simulink model "Robocon_mark1_1"  (R2020b)
settings: Solver=ode45  StartTime=0.0  StopTime=10.0  MaxStep=1e-2  RelTol=1e-4  AbsTol=1e-5  EnableMultiTasking=on
values from neighbouring files (symbols this model uses):
  arena_breadth = 10    [Robocon_DataFile.m]
  arena_length = 13.3    [Robocon_DataFile.m]
undefined symbols (not defined in the file or in its folder): DiscIntNeverNeededParam, sigbuilder_block, smiData, X, Y, Z
libraries: sm_lib x232, Contact_Forces_Lib x55, nesl_utility x9, mobileRoboticsLib x4, simulink_extras x2, fl_lib x1
(part 6 of 6)

== system Robocon_mark1_1/TR ROBOT/CONTACT FORCE/PLATE CONTACT4 ==
  Sphere to Plane Force : Contact_Forces_Lib/3D/Sphere to Plane Force  sphere_rad=rugby_main  plane_lenx=0.16  plane_leny=0.191  plane_depth=0  force_law=Linear  k_contact=1e4  b_contact=1e2  pen_full_damp_F=1e-4  pen_exponent=1  custom_param_1=1  custom_param_2=1  friction_law=Stick-Slip Continuous  mu_kinetic=0.5  mu_static=0.7  v_thr=0.001  vis_on=off  vis_opc_en=0  vis_len_plaBz=0.005  vis_clr=[0.9 0.2 0.2]  vis_opc=0.7
  Terminator1 : Terminator
  MIDDLE : PMIOPort  Side=Left
  TO PLATE : PMIOPort  Port=2  Side=Right
  wires:
  Sphere to Plane Force/1 -> Terminator1/1
  connections:
  TO PLATE/RConn1 -- Sphere to Plane Force/RConn1
  Sphere to Plane Force/LConn1 -- MIDDLE/RConn1

== system Robocon_mark1_1/TR ROBOT/CONTACT FORCE/PLATE CONTACT5 ==
  Sphere to Plane Force : Contact_Forces_Lib/3D/Sphere to Plane Force  sphere_rad=rugby_main  plane_lenx=0.16  plane_leny=0.097  plane_depth=0  force_law=Linear  k_contact=1e4  b_contact=1e2  pen_full_damp_F=1e-4  pen_exponent=1  custom_param_1=1  custom_param_2=1  friction_law=Stick-Slip Continuous  mu_kinetic=0.5  mu_static=0.7  v_thr=0.001  vis_on=off  vis_opc_en=0  vis_len_plaBz=0.005  vis_clr=[0.9 0.2 0.2]  vis_opc=0.7
  Sphere to Plane Force1 : Contact_Forces_Lib/3D/Sphere to Plane Force  sphere_rad=rugby_middle_lower  plane_lenx=0.16  plane_leny=0.097  plane_depth=0  force_law=Linear  k_contact=1e4  b_contact=1e2  pen_full_damp_F=1e-4  pen_exponent=1  custom_param_1=1  custom_param_2=1  friction_law=Stick-Slip Continuous  mu_kinetic=0.5  mu_static=0.7  v_thr=0.001  vis_on=off  vis_opc_en=0  vis_len_plaBz=0.005  vis_clr=[0.9 0.2 0.2]  vis_opc=0.7
  Sphere to Plane Force2 : Contact_Forces_Lib/3D/Sphere to Plane Force  sphere_rad=rugby_middle_upper  plane_lenx=0.16  plane_leny=0.097  plane_depth=0  force_law=Linear  k_contact=1e4  b_contact=1e2  pen_full_damp_F=1e-4  pen_exponent=1  custom_param_1=1  custom_param_2=1  friction_law=Stick-Slip Continuous  mu_kinetic=0.5  mu_static=0.7  v_thr=0.001  vis_on=off  vis_opc_en=0  vis_len_plaBz=0.005  vis_clr=[0.9 0.2 0.2]  vis_opc=0.7
  Terminator : Terminator
  Terminator1 : Terminator
  Terminator2 : Terminator
  "UPPER " : PMIOPort  Side=Left
  MIDDLE : PMIOPort  Port=2  Side=Left
  TO PLATE : PMIOPort  Port=3  Side=Right
  LOWER : PMIOPort  Port=4  Side=Left
  wires:
  Sphere to Plane Force2/1 -> Terminator/1
  Sphere to Plane Force1/1 -> Terminator2/1
  Sphere to Plane Force/1 -> Terminator1/1
  connections:
  Sphere to Plane Force/LConn1 -- MIDDLE/RConn1
  Sphere to Plane Force1/LConn1 -- LOWER/RConn1
  Sphere to Plane Force2/LConn1 -- "UPPER "/RConn1
  TO PLATE/RConn1 -- Sphere to Plane Force2/RConn1 -- Sphere to Plane Force/RConn1 -- Sphere to Plane Force1/RConn1

== system Robocon_mark1_1/TR ROBOT/CONTACT FORCE/ROUND PLATE CONTACT ==
  Sphere to Tube Force : Contact_Forces_Lib/3D/Sphere to Tube Force  radius_sphere=rugby_middle_upper  radius_tube=0.188  d_tube=0.01  l_tube=0.16  active_angle=[-27 87]  force_law=Linear  k_contact=1e6  b_contact=1e2  pen_full_damp_F=1e-4  pen_exponent=1  custom_param_1=1  custom_param_2=1  friction_law=Stick-Slip Continuous  mu_kinetic=0.5  mu_static=0.7  v_thr=0.001  vis_on=off  vis_opc_en=0  vis_len_tubBx=0.225*0.02  vis_clr=[0.9 0.2 0.2]  vis_opc=0.7
      settings: SourceProductName=Simscape Multibody Contact Forces Library
  Sphere to Tube Force1 : Contact_Forces_Lib/3D/Sphere to Tube Force  radius_sphere=rugby_main  radius_tube=0.188  d_tube=0.01  l_tube=0.16  active_angle=[-27 87]  force_law=Linear  k_contact=1e3  b_contact=1e2  pen_full_damp_F=1e-4  pen_exponent=1  custom_param_1=1  custom_param_2=1  friction_law=Stick-Slip Continuous  mu_kinetic=0.5  mu_static=0.7  v_thr=0.001  vis_on=off  vis_opc_en=0  vis_len_tubBx=0.225*0.02  vis_clr=[0.9 0.2 0.2]  vis_opc=0.7
      settings: SourceProductName=Simscape Multibody Contact Forces Library
  Sphere to Tube Force2 : Contact_Forces_Lib/3D/Sphere to Tube Force  radius_sphere=rugby_middle_lower  radius_tube=0.188  d_tube=0.01  l_tube=0.16  active_angle=[-27 87]  force_law=Linear  k_contact=1e6  b_contact=1e2  pen_full_damp_F=1e-4  pen_exponent=1  custom_param_1=1  custom_param_2=1  friction_law=Stick-Slip Continuous  mu_kinetic=0.5  mu_static=0.7  v_thr=0.001  vis_on=off  vis_opc_en=0  vis_len_tubBx=0.225*0.02  vis_clr=[0.9 0.2 0.2]  vis_opc=0.7
      settings: SourceProductName=Simscape Multibody Contact Forces Library
  Terminator : Terminator
  Terminator1 : Terminator
  Terminator2 : Terminator
  "UPPER " : PMIOPort  Side=Left
  MIDDLE : PMIOPort  Port=2  Side=Left
  TO PLATE : PMIOPort  Port=3  Side=Right
  LOWER : PMIOPort  Port=4  Side=Left
  wires:
  Sphere to Tube Force1/1 -> Terminator1/1
  Sphere to Tube Force2/1 -> Terminator2/1
  Sphere to Tube Force/1 -> Terminator/1
  connections:
  Sphere to Tube Force/RConn1 -- TO PLATE/RConn1 -- Sphere to Tube Force1/RConn1 -- Sphere to Tube Force2/RConn1
  "UPPER "/RConn1 -- Sphere to Tube Force/LConn1
  Sphere to Tube Force2/LConn1 -- LOWER/RConn1
  Sphere to Tube Force1/LConn1 -- MIDDLE/RConn1

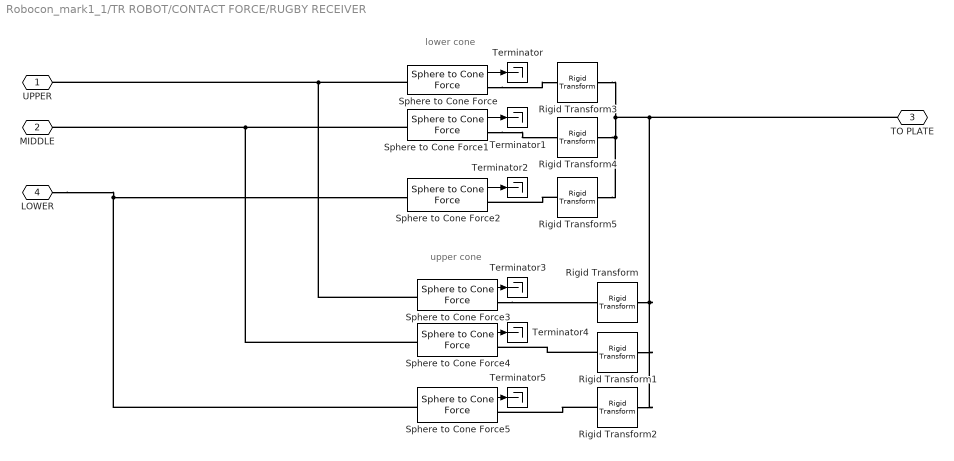
== system Robocon_mark1_1/TR ROBOT/CONTACT FORCE/RUGBY RECEIVER ==
  note: lower cone
  note: upper cone
  Rigid Transform : sm_lib/Frames and Transforms/Rigid Transform  TranslationMethod=StandardAxis  TranslationStandardOffset=710  TranslationLengthUnit=mm  TranslationStandardAxis=-Z  TranslationCartesianOffset=[0 0 0]  TranslationROffset=0  TranslationROffsetUnits=m  TranslationZOffset=0  TranslationZOffsetUnits=m  TranslationThetaOffset=0  TranslationThetaOffsetUnits=deg  RotationMethod=StandardAxis  RotationAngleUnits=deg  RotationStandardAxis=+Z  RotationAngle=-30  RotationArbitraryAxis=[0 0 1]  FollAlignAxisA=+X  BaseAlignAxisA=+Y  FollAlignAxisB=+Y  BaseAlignAxisB=+Z  RotationSequenceAxes=FollowerAxes  RotationSequence=XYX  RotationSequenceAngles=[0 0 0]  RotationSequenceAnglesUnits=deg  RotationMatrix=[1 0 0; 0 1 0; 0 0 1]
  Rigid Transform1 : sm_lib/Frames and Transforms/Rigid Transform  TranslationMethod=StandardAxis  TranslationStandardOffset=710  TranslationLengthUnit=mm  TranslationStandardAxis=-Z  TranslationCartesianOffset=[0 0 0]  TranslationROffset=0  TranslationROffsetUnits=m  TranslationZOffset=0  TranslationZOffsetUnits=m  TranslationThetaOffset=0  TranslationThetaOffsetUnits=deg  RotationMethod=StandardAxis  RotationAngleUnits=deg  RotationStandardAxis=+Z  RotationAngle=-30  RotationArbitraryAxis=[0 0 1]  FollAlignAxisA=+X  BaseAlignAxisA=+Y  FollAlignAxisB=+Y  BaseAlignAxisB=+Z  RotationSequenceAxes=FollowerAxes  RotationSequence=XYX  RotationSequenceAngles=[0 0 0]  RotationSequenceAnglesUnits=deg  RotationMatrix=[1 0 0; 0 1 0; 0 0 1]
  Rigid Transform2 : sm_lib/Frames and Transforms/Rigid Transform  TranslationMethod=StandardAxis  TranslationStandardOffset=710  TranslationLengthUnit=mm  TranslationStandardAxis=-Z  TranslationCartesianOffset=[0 0 0]  TranslationROffset=0  TranslationROffsetUnits=m  TranslationZOffset=0  TranslationZOffsetUnits=m  TranslationThetaOffset=0  TranslationThetaOffsetUnits=deg  RotationMethod=StandardAxis  RotationAngleUnits=deg  RotationStandardAxis=+Z  RotationAngle=-30  RotationArbitraryAxis=[0 0 1]  FollAlignAxisA=+X  BaseAlignAxisA=+Y  FollAlignAxisB=+Y  BaseAlignAxisB=+Z  RotationSequenceAxes=FollowerAxes  RotationSequence=XYX  RotationSequenceAngles=[0 0 0]  RotationSequenceAnglesUnits=deg  RotationMatrix=[1 0 0; 0 1 0; 0 0 1]
  Rigid Transform3 : sm_lib/Frames and Transforms/Rigid Transform  TranslationMethod=StandardAxis  TranslationStandardOffset=345  TranslationLengthUnit=mm  TranslationStandardAxis=-Z  TranslationCartesianOffset=[0 0 0]  TranslationROffset=0  TranslationROffsetUnits=m  TranslationZOffset=0  TranslationZOffsetUnits=m  TranslationThetaOffset=0  TranslationThetaOffsetUnits=deg  RotationMethod=StandardAxis  RotationAngleUnits=deg  RotationStandardAxis=+Z  RotationAngle=150  RotationArbitraryAxis=[0 0 1]  FollAlignAxisA=+X  BaseAlignAxisA=+Y  FollAlignAxisB=+Y  BaseAlignAxisB=+Z  RotationSequenceAxes=FollowerAxes  RotationSequence=XYX  RotationSequenceAngles=[0 0 0]  RotationSequenceAnglesUnits=deg  RotationMatrix=[1 0 0; 0 1 0; 0 0 1]
  Rigid Transform4 : sm_lib/Frames and Transforms/Rigid Transform  TranslationMethod=StandardAxis  TranslationStandardOffset=345  TranslationLengthUnit=mm  TranslationStandardAxis=-Z  TranslationCartesianOffset=[0 0 0]  TranslationROffset=0  TranslationROffsetUnits=m  TranslationZOffset=0  TranslationZOffsetUnits=m  TranslationThetaOffset=0  TranslationThetaOffsetUnits=deg  RotationMethod=StandardAxis  RotationAngleUnits=deg  RotationStandardAxis=+Z  RotationAngle=150  RotationArbitraryAxis=[0 0 1]  FollAlignAxisA=+X  BaseAlignAxisA=+Y  FollAlignAxisB=+Y  BaseAlignAxisB=+Z  RotationSequenceAxes=FollowerAxes  RotationSequence=XYX  RotationSequenceAngles=[0 0 0]  RotationSequenceAnglesUnits=deg  RotationMatrix=[1 0 0; 0 1 0; 0 0 1]
  Rigid Transform5 : sm_lib/Frames and Transforms/Rigid Transform  TranslationMethod=StandardAxis  TranslationStandardOffset=345  TranslationLengthUnit=mm  TranslationStandardAxis=-Z  TranslationCartesianOffset=[0 0 0]  TranslationROffset=0  TranslationROffsetUnits=m  TranslationZOffset=0  TranslationZOffsetUnits=m  TranslationThetaOffset=0  TranslationThetaOffsetUnits=deg  RotationMethod=StandardAxis  RotationAngleUnits=deg  RotationStandardAxis=+Z  RotationAngle=150  RotationArbitraryAxis=[0 0 1]  FollAlignAxisA=+X  BaseAlignAxisA=+Y  FollAlignAxisB=+Y  BaseAlignAxisB=+Z  RotationSequenceAxes=FollowerAxes  RotationSequence=XYX  RotationSequenceAngles=[0 0 0]  RotationSequenceAnglesUnits=deg  RotationMatrix=[1 0 0; 0 1 0; 0 0 1]
  Sphere to Cone Force : Contact_Forces_Lib/3D/Sphere to Cone Force  radius_sphere=rugby_middle_upper  cone_or=0.2  cone_ir=0.2  cone_theta=80  cone_h=0.345  active_angle=[-90 90]  d_cone=0  r_cone=0  cosConeTh=0  sinConeTh=0  force_law=Linear  k_contact=1e3  b_contact=100  pen_full_damp_F=1e-4  pen_exponent=1  custom_param_1=1  custom_param_2=1  friction_law=Stick-Slip Continuous  mu_kinetic=0.5  mu_static=0.7  v_thr=0.001  vis_on=off  vis_opc_en=0  vis_depth_conBx=0.02  vis_clr=[0.9 0.2 0.2]  vis_opc=0.7
      settings: SourceProductName=Simscape Multibody Contact Forces Library
  Sphere to Cone Force1 : Contact_Forces_Lib/3D/Sphere to Cone Force  radius_sphere=rugby_main  cone_or=0.2  cone_ir=0.2  cone_theta=80  cone_h=0.345  active_angle=[-90 90]  d_cone=0  r_cone=0  cosConeTh=0  sinConeTh=0  force_law=Linear  k_contact=1e3  b_contact=100  pen_full_damp_F=1e-4  pen_exponent=1  custom_param_1=1  custom_param_2=1  friction_law=Stick-Slip Continuous  mu_kinetic=0.5  mu_static=0.7  v_thr=0.001  vis_on=off  vis_opc_en=0  vis_depth_conBx=0.02  vis_clr=[0.9 0.2 0.2]  vis_opc=0.7
      settings: SourceProductName=Simscape Multibody Contact Forces Library
  Sphere to Cone Force2 : Contact_Forces_Lib/3D/Sphere to Cone Force  radius_sphere=rugby_middle_lower  cone_or=0.2  cone_ir=0.2  cone_theta=80  cone_h=0.345  active_angle=[-90 90]  d_cone=0  r_cone=0  cosConeTh=0  sinConeTh=0  force_law=Linear  k_contact=1e3  b_contact=1e2  pen_full_damp_F=1e-4  pen_exponent=1  custom_param_1=1  custom_param_2=1  friction_law=Stick-Slip Continuous  mu_kinetic=0.5  mu_static=0.7  v_thr=0.001  vis_on=off  vis_opc_en=0  vis_depth_conBx=0.02  vis_clr=[0.9 0.2 0.2]  vis_opc=0.7
      settings: SourceProductName=Simscape Multibody Contact Forces Library
  Sphere to Cone Force3 : Contact_Forces_Lib/3D/Sphere to Cone Force  radius_sphere=rugby_middle_upper  cone_or=0.27  cone_ir=0.27  cone_theta=80  cone_h=0.71  active_angle=[-90 90]  d_cone=0  r_cone=0  cosConeTh=0  sinConeTh=0  force_law=Linear  k_contact=1e3  b_contact=1e2  pen_full_damp_F=1e-4  pen_exponent=1  custom_param_1=1  custom_param_2=1  friction_law=Stick-Slip Continuous  mu_kinetic=0.5  mu_static=0.7  v_thr=0.001  vis_on=off  vis_opc_en=0  vis_depth_conBx=0.02  vis_clr=[0.9 0.2 0.2]  vis_opc=0.7
      settings: SourceProductName=Simscape Multibody Contact Forces Library
  Sphere to Cone Force4 : Contact_Forces_Lib/3D/Sphere to Cone Force  radius_sphere=rugby_main  cone_or=0.27  cone_ir=0.27  cone_theta=80  cone_h=0.71  active_angle=[-90 90]  d_cone=0  r_cone=0  cosConeTh=0  sinConeTh=0  force_law=Linear  k_contact=1e3  b_contact=1e2  pen_full_damp_F=1e-4  pen_exponent=1  custom_param_1=1  custom_param_2=1  friction_law=Stick-Slip Continuous  mu_kinetic=0.5  mu_static=0.7  v_thr=0.001  vis_on=off  vis_opc_en=0  vis_depth_conBx=0.02  vis_clr=[0.9 0.2 0.2]  vis_opc=0.7
      settings: SourceProductName=Simscape Multibody Contact Forces Library
  Sphere to Cone Force5 : Contact_Forces_Lib/3D/Sphere to Cone Force  radius_sphere=rugby_middle_lower  cone_or=0.27  cone_ir=0.27  cone_theta=80  cone_h=0.71  active_angle=[-90 90]  d_cone=0  r_cone=0  cosConeTh=0  sinConeTh=0  force_law=Linear  k_contact=1e3  b_contact=1e2  pen_full_damp_F=1e-4  pen_exponent=1  custom_param_1=1  custom_param_2=1  friction_law=Stick-Slip Continuous  mu_kinetic=0.5  mu_static=0.7  v_thr=0.001  vis_on=off  vis_opc_en=0  vis_depth_conBx=0.02  vis_clr=[0.9 0.2 0.2]  vis_opc=0.7
      settings: SourceProductName=Simscape Multibody Contact Forces Library
  Terminator{,1..5} (6 alike) : Terminator
  "UPPER " : PMIOPort  Side=Left
  MIDDLE : PMIOPort  Port=2  Side=Left
  TO PLATE : PMIOPort  Port=3  Side=Right
  LOWER : PMIOPort  Port=4  Side=Left
  wires:
  Sphere to Cone Force/1 -> Terminator/1
  Sphere to Cone Force2/1 -> Terminator2/1
  Sphere to Cone Force1/1 -> Terminator1/1
  Sphere to Cone Force3/1 -> Terminator3/1
  Sphere to Cone Force4/1 -> Terminator4/1
  Sphere to Cone Force5/1 -> Terminator5/1
  connections:
  Sphere to Cone Force1/LConn1 -- Sphere to Cone Force4/LConn1 -- MIDDLE/RConn1
  LOWER/RConn1 -- Sphere to Cone Force5/LConn1 -- Sphere to Cone Force2/LConn1
  Sphere to Cone Force/LConn1 -- Sphere to Cone Force3/LConn1 -- "UPPER "/RConn1
  Sphere to Cone Force3/RConn1 -- Rigid Transform/RConn1
  Rigid Transform2/RConn1 -- Sphere to Cone Force5/RConn1
  Rigid Transform1/RConn1 -- Sphere to Cone Force4/RConn1
  Rigid Transform/LConn1 -- Rigid Transform1/LConn1 -- Rigid Transform2/LConn1 -- Rigid Transform3/LConn1 -- Rigid Transform5/LConn1 -- Rigid Transform4/LConn1 -- TO PLATE/RConn1
  Sphere to Cone Force/RConn1 -- Rigid Transform3/RConn1
  Sphere to Cone Force1/RConn1 -- Rigid Transform4/RConn1
  Rigid Transform5/RConn1 -- Sphere to Cone Force2/RConn1

== system Robocon_mark1_1/TR ROBOT/trleftgripper_1_RIGID1/Signal Builder ==
  Demux : Demux  Tag=STV Demux  Outputs=1
      settings: DisplayOption=none
  FromWs : FromWorkspace  Tag=STV FromWs  VariableName=tuvar
      SigBuilderData=|
      | common.afterFinalStr = 'Extrapolate'
      | common.sampleTime = 0
      | dataSet.timeRange = [0 30]
      | dataSet.name = 'Group 1'
      | sbobj.Groups.Name = 'Group 1'
      | sbobj.Groups.Signals.Name = 'Signal 1'
      | sbobj.Groups.Signals.XData = [0 12.95 12.95 30]
      | sbobj.Groups.Signals.YData = [0 0 1 1]
      | sbobj.Groups.TimeRange = [0 30]
  Signal 1 : Outport  Tag=STV Outport
  wires:
  Demux/1 -> Signal 1/1
  FromWs/1 -> Demux/1

== system Robocon_mark1_1/PR Robot/SPOON/CONTACT FORCES/Subsystem1 ==
  Sphere to Plane Force1 : Contact_Forces_Lib/3D/Sphere to Plane Force  sphere_rad=rugby_main  plane_lenx=0.29  plane_leny=0.15  plane_depth=0  force_law=Linear  k_contact=400000  b_contact=250  pen_full_damp_F=1e-2  pen_exponent=2  custom_param_1=1  custom_param_2=1  friction_law=Stick-Slip Continuous  mu_kinetic=0.5  mu_static=0.7  v_thr=0.001  vis_on=off  vis_opc_en=0  vis_len_plaBz=0.005  vis_clr=[0.9 0.2 0.2]  vis_opc=0.7
  Sphere to Plane Force2 : Contact_Forces_Lib/3D/Sphere to Plane Force  sphere_rad=rugby_middle_lower  plane_lenx=0.29  plane_leny=0.15  plane_depth=0  force_law=Linear  k_contact=1000  b_contact=50  pen_full_damp_F=1e-2  pen_exponent=2  custom_param_1=1  custom_param_2=1  friction_law=Stick-Slip Continuous  mu_kinetic=0.5  mu_static=0.7  v_thr=0.001  vis_on=off  vis_opc_en=0  vis_len_plaBz=0.005  vis_clr=[0.9 0.2 0.2]  vis_opc=0.7
  Sphere to Plane Force6 : Contact_Forces_Lib/3D/Sphere to Plane Force  sphere_rad=rugby_middle_upper  plane_lenx=0.29  plane_leny=0.15  plane_depth=0  force_law=Linear  k_contact=1000  b_contact=50  pen_full_damp_F=1e-2  pen_exponent=2  custom_param_1=1  custom_param_2=1  friction_law=Stick-Slip Continuous  mu_kinetic=0.5  mu_static=0.7  v_thr=0.001  vis_on=off  vis_opc_en=0  vis_len_plaBz=0.005  vis_clr=[0.9 0.2 0.2]  vis_opc=0.7
  Terminator6 : Terminator
  Terminator7 : Terminator
  Terminator8 : Terminator
  Conn1 : PMIOPort  Side=Left
  upper : PMIOPort  Port=2  Side=Left
  middle : PMIOPort  Port=3  Side=Left
  lower : PMIOPort  Port=4  Side=Left
  wires:
  Sphere to Plane Force6/1 -> Terminator6/1
  Sphere to Plane Force1/1 -> Terminator7/1
  Sphere to Plane Force2/1 -> Terminator8/1
  connections:
  Sphere to Plane Force2/LConn1 -- lower/RConn1
  Sphere to Plane Force1/LConn1 -- middle/RConn1
  Sphere to Plane Force6/LConn1 -- upper/RConn1
  Conn1/RConn1 -- Sphere to Plane Force6/RConn1 -- Sphere to Plane Force2/RConn1 -- Sphere to Plane Force1/RConn1

== system Robocon_mark1_1/PR Robot/SPOON/CONTACT FORCES/Subsystem2 ==
  Sphere to Plane Force1 : Contact_Forces_Lib/3D/Sphere to Plane Force  sphere_rad=rugby_main  plane_lenx=0.28  plane_leny=0.17  plane_depth=0  force_law=Linear  k_contact=10000  b_contact=200  pen_full_damp_F=1e-2  pen_exponent=2  custom_param_1=1  custom_param_2=1  friction_law=Stick-Slip Continuous  mu_kinetic=0.5  mu_static=0.7  v_thr=0.001  vis_on=off  vis_opc_en=0  vis_len_plaBz=0.005  vis_clr=[0.9 0.2 0.2]  vis_opc=0.7
  Sphere to Plane Force2 : Contact_Forces_Lib/3D/Sphere to Plane Force  sphere_rad=rugby_middle_lower  plane_lenx=0.28  plane_leny=0.17  plane_depth=0  force_law=Nonlinear  k_contact=400  b_contact=50  pen_full_damp_F=1e-2  pen_exponent=2  custom_param_1=1  custom_param_2=1  friction_law=Stick-Slip Continuous  mu_kinetic=0.5  mu_static=0.7  v_thr=0.001  vis_on=off  vis_opc_en=0  vis_len_plaBz=0.005  vis_clr=[0.9 0.2 0.2]  vis_opc=0.7
  Sphere to Plane Force6 : Contact_Forces_Lib/3D/Sphere to Plane Force  sphere_rad=rugby_middle_upper  plane_lenx=0.28  plane_leny=0.17  plane_depth=0  force_law=Nonlinear  k_contact=400  b_contact=50  pen_full_damp_F=1e-2  pen_exponent=2  custom_param_1=1  custom_param_2=1  friction_law=Stick-Slip Continuous  mu_kinetic=0.5  mu_static=0.7  v_thr=0.001  vis_on=off  vis_opc_en=0  vis_len_plaBz=0.005  vis_clr=[0.9 0.2 0.2]  vis_opc=0.7
  Terminator6 : Terminator
  Terminator7 : Terminator
  Terminator8 : Terminator
  Conn1 : PMIOPort  Side=Left
  upper : PMIOPort  Port=2  Side=Left
  middle : PMIOPort  Port=3  Side=Left
  lower : PMIOPort  Port=4  Side=Left
  wires:
  Sphere to Plane Force2/1 -> Terminator8/1
  Sphere to Plane Force1/1 -> Terminator7/1
  Sphere to Plane Force6/1 -> Terminator6/1
  connections:
  Conn1/RConn1 -- Sphere to Plane Force6/RConn1 -- Sphere to Plane Force2/RConn1 -- Sphere to Plane Force1/RConn1
  Sphere to Plane Force6/LConn1 -- upper/RConn1
  Sphere to Plane Force1/LConn1 -- middle/RConn1
  Sphere to Plane Force2/LConn1 -- lower/RConn1

== system Robocon_mark1_1/PR Robot/SPOON/CONTACT FORCES/Subsystem3 ==
  Sphere to Plane Force1 : Contact_Forces_Lib/3D/Sphere to Plane Force  sphere_rad=rugby_main  plane_lenx=0.17  plane_leny=0.15  plane_depth=0  force_law=Linear  k_contact=400000  b_contact=250  pen_full_damp_F=1e-2  pen_exponent=2  custom_param_1=1  custom_param_2=1  friction_law=Stick-Slip Continuous  mu_kinetic=0.5  mu_static=0.7  v_thr=0.001  vis_on=off  vis_opc_en=0  vis_len_plaBz=0.005  vis_clr=[0.9 0.2 0.2]  vis_opc=0.7
  Sphere to Plane Force2 : Contact_Forces_Lib/3D/Sphere to Plane Force  sphere_rad=rugby_middle_upper  plane_lenx=0.17  plane_leny=0.15  plane_depth=0  force_law=Linear  k_contact=400000  b_contact=250  pen_full_damp_F=1e-2  pen_exponent=2  custom_param_1=1  custom_param_2=1  friction_law=Stick-Slip Continuous  mu_kinetic=0.5  mu_static=0.7  v_thr=0.001  vis_on=off  vis_opc_en=0  vis_len_plaBz=0.005  vis_clr=[0.9 0.2 0.2]  vis_opc=0.7
  Sphere to Plane Force6 : Contact_Forces_Lib/3D/Sphere to Plane Force  sphere_rad=rugby_middle_lower  plane_lenx=0.17  plane_leny=0.15  plane_depth=0  force_law=Linear  k_contact=400000  b_contact=250  pen_full_damp_F=1e-2  pen_exponent=2  custom_param_1=1  custom_param_2=1  friction_law=Stick-Slip Continuous  mu_kinetic=0.5  mu_static=0.7  v_thr=0.001  vis_on=off  vis_opc_en=0  vis_len_plaBz=0.005  vis_clr=[0.9 0.2 0.2]  vis_opc=0.7
  Terminator6 : Terminator
  Terminator7 : Terminator
  Terminator8 : Terminator
  Conn1 : PMIOPort  Side=Left
  upper : PMIOPort  Port=2  Side=Left
  middle : PMIOPort  Port=3  Side=Left
  lower : PMIOPort  Port=4  Side=Left
  wires:
  Sphere to Plane Force2/1 -> Terminator6/1
  Sphere to Plane Force1/1 -> Terminator7/1
  Sphere to Plane Force6/1 -> Terminator8/1
  connections:
  Sphere to Plane Force6/LConn1 -- lower/RConn1
  Sphere to Plane Force1/LConn1 -- middle/RConn1
  Sphere to Plane Force2/LConn1 -- upper/RConn1
  Conn1/RConn1 -- Sphere to Plane Force2/RConn1 -- Sphere to Plane Force1/RConn1 -- Sphere to Plane Force6/RConn1

== system Robocon_mark1_1/PR Robot/SPOON/CONTACT FORCES/Subsystem4 ==
  Sphere to Plane Force1 : Contact_Forces_Lib/3D/Sphere to Plane Force  sphere_rad=rugby_main  plane_lenx=0.29  plane_leny=0.15  plane_depth=0  force_law=Linear  k_contact=400000  b_contact=250  pen_full_damp_F=1e-2  pen_exponent=2  custom_param_1=1  custom_param_2=1  friction_law=Stick-Slip Continuous  mu_kinetic=0.5  mu_static=0.7  v_thr=0.001  vis_on=off  vis_opc_en=0  vis_len_plaBz=0.005  vis_clr=[0.9 0.2 0.2]  vis_opc=0.7
  Sphere to Plane Force2 : Contact_Forces_Lib/3D/Sphere to Plane Force  sphere_rad=rugby_middle_lower  plane_lenx=0.29  plane_leny=0.15  plane_depth=0  force_law=Linear  k_contact=1000  b_contact=50  pen_full_damp_F=1e-2  pen_exponent=2  custom_param_1=1  custom_param_2=1  friction_law=Stick-Slip Continuous  mu_kinetic=0.5  mu_static=0.7  v_thr=0.001  vis_on=off  vis_opc_en=0  vis_len_plaBz=0.005  vis_clr=[0.9 0.2 0.2]  vis_opc=0.7
  Sphere to Plane Force6 : Contact_Forces_Lib/3D/Sphere to Plane Force  sphere_rad=rugby_middle_upper  plane_lenx=0.29  plane_leny=0.15  plane_depth=0  force_law=Linear  k_contact=1000  b_contact=50  pen_full_damp_F=1e-1  pen_exponent=2  custom_param_1=1  custom_param_2=1  friction_law=Stick-Slip Continuous  mu_kinetic=0.5  mu_static=0.7  v_thr=0.001  vis_on=off  vis_opc_en=0  vis_len_plaBz=0.005  vis_clr=[0.9 0.2 0.2]  vis_opc=0.7
  Terminator6 : Terminator
  Terminator7 : Terminator
  Terminator8 : Terminator
  Conn1 : PMIOPort  Side=Left
  upper : PMIOPort  Port=2  Side=Left
  middle : PMIOPort  Port=3  Side=Left
  lower : PMIOPort  Port=4  Side=Left
  wires:
  Sphere to Plane Force2/1 -> Terminator8/1
  Sphere to Plane Force1/1 -> Terminator7/1
  Sphere to Plane Force6/1 -> Terminator6/1
  connections:
  Sphere to Plane Force6/RConn1 -- Conn1/RConn1 -- Sphere to Plane Force2/RConn1 -- Sphere to Plane Force1/RConn1
  Sphere to Plane Force6/LConn1 -- upper/RConn1
  Sphere to Plane Force1/LConn1 -- middle/RConn1
  Sphere to Plane Force2/LConn1 -- lower/RConn1

== system Robocon_mark1_1/PR Robot/SPOON/CONTACT FORCES/Subsystem5 ==
  Sphere to Plane Force1 : Contact_Forces_Lib/3D/Sphere to Plane Force  sphere_rad=rugby_main  plane_lenx=0.17  plane_leny=0.15  plane_depth=0  force_law=Nonlinear  k_contact=400000  b_contact=250  pen_full_damp_F=1e-2  pen_exponent=2  custom_param_1=1  custom_param_2=1  friction_law=Stick-Slip Continuous  mu_kinetic=0.5  mu_static=0.7  v_thr=0.001  vis_on=off  vis_opc_en=0  vis_len_plaBz=0.005  vis_clr=[0.9 0.2 0.2]  vis_opc=0.7
  Sphere to Plane Force2 : Contact_Forces_Lib/3D/Sphere to Plane Force  sphere_rad=rugby_middle_lower  plane_lenx=0.17  plane_leny=0.15  plane_depth=0  force_law=Linear  k_contact=400000  b_contact=250  pen_full_damp_F=1e-2  pen_exponent=2  custom_param_1=1  custom_param_2=1  friction_law=Stick-Slip Continuous  mu_kinetic=0.5  mu_static=0.7  v_thr=0.001  vis_on=off  vis_opc_en=0  vis_len_plaBz=0.005  vis_clr=[0.9 0.2 0.2]  vis_opc=0.7
  Sphere to Plane Force6 : Contact_Forces_Lib/3D/Sphere to Plane Force  sphere_rad=rugby_middle_upper  plane_lenx=0.17  plane_leny=0.15  plane_depth=0  force_law=Linear  k_contact=400000  b_contact=250  pen_full_damp_F=1e-2  pen_exponent=2  custom_param_1=1  custom_param_2=1  friction_law=Stick-Slip Continuous  mu_kinetic=0.5  mu_static=0.7  v_thr=0.001  vis_on=off  vis_opc_en=0  vis_len_plaBz=0.005  vis_clr=[0.9 0.2 0.2]  vis_opc=0.7
  Terminator6 : Terminator
  Terminator7 : Terminator
  Terminator8 : Terminator
  Conn1 : PMIOPort  Side=Left
  upper : PMIOPort  Port=2  Side=Left
  middle : PMIOPort  Port=3  Side=Left
  lower : PMIOPort  Port=4  Side=Left
  wires:
  Sphere to Plane Force2/1 -> Terminator8/1
  Sphere to Plane Force1/1 -> Terminator7/1
  Sphere to Plane Force6/1 -> Terminator6/1
  connections:
  Sphere to Plane Force6/RConn1 -- Conn1/RConn1 -- Sphere to Plane Force2/RConn1 -- Sphere to Plane Force1/RConn1
  Sphere to Plane Force6/LConn1 -- upper/RConn1
  Sphere to Plane Force1/LConn1 -- middle/RConn1
  Sphere to Plane Force2/LConn1 -- lower/RConn1
